simulink model "OilWellDrillingTesting"  (R2021a)
settings: Solver=ode4  StartTime=0.0  StopTime=4800  FixedStep=0.1  RelTol=1e-3
libraries: simulink x1
settings Model: Creator=isak.skeie  LastModifiedBy=isak.skeie

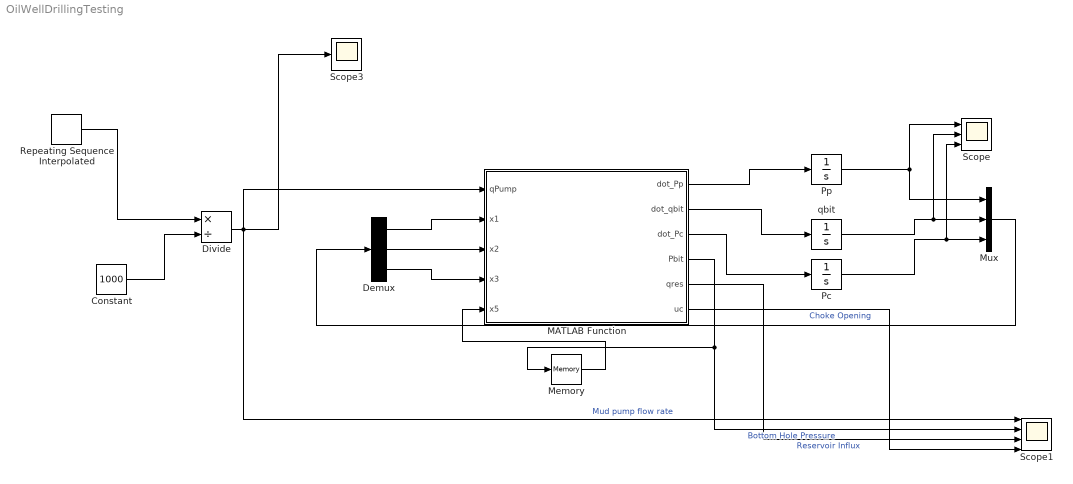
== system OilWellDrillingTesting ==
  Constant : Constant  Value=1000
  Demux : Demux  Outputs=3
  Divide : Product  Inputs=*/
  MATLAB Function : MATLAB Function  TreatAsAtomicUnit=on
  Memory : Memory
  Mux : Mux  Inputs=3
  Pc : Integrator  InitialCondition=5*10^5
  Pp : Integrator  InitialCondition=8*10^5
  Repeating Sequence Interpolated : simulink/Sources/Repeating Sequence Interpolated  OutValues="[25 25  0 0  25 25 0 0 25 25].'"  TimeValues=[0 600 900 1500 1800 2700 3000 3600 3900 4800].'  LookUpMeth=Interpolation-Use End Values  tsamp=0.1  OutMin=[0]  OutMax=[0.025]  OutDataTypeStr=double  OutputDataTypeScalingMode=double  OutDataType=fixdt(0,8)  OutScaling=2^-10
  Scope : Scope  NumInputPorts=3
  Scope1 : Scope  NumInputPorts=4
  Scope3 : Scope
  qbit : Integrator  InitialCondition=0.025
  wires:
  MATLAB Function/1(dot_Pp) -> Pp/1
  MATLAB Function/2(dot_qbit) -> qbit/1
  MATLAB Function/3(dot_Pc) -> Pc/1
  Pp/1 -> Mux/1, Scope/1
  qbit/1 -> Scope/2, Mux/2
  Pc/1 -> Scope/3, Mux/3
  Demux/1 -> MATLAB Function/2(x1)
  Demux/2 -> MATLAB Function/3(x2)
  Demux/3 -> MATLAB Function/4(x3)
  Mux/1 -> Demux/1
  MATLAB Function/4(Pbit) -> Scope1/2, Memory/1  "Bottom Hole Pressure"
  Memory/1 -> MATLAB Function/5(x5)
  Repeating Sequence Interpolated/1 -> Divide/1
  Constant/1 -> Divide/2
  Divide/1 -> Scope1/1, MATLAB Function/1(qPump), Scope3/1  "Mud pump flow rate"
  MATLAB Function/5(qres) -> Scope1/3  "Reservoir Influx"
  MATLAB Function/6(uc) -> Scope1/4  "Choke Opening"

== matlab function OilWellDrillingTesting/MATLAB Function ==
  data: qPump input; x1 input; dot_Pp output; x2 input; x3 input; dot_qbit output; dot_Pc output; Pbit output; qres output; x5 input; uc output
function [dot_Pp, dot_qbit, dot_Pc,Pbit, qres, uc] = OilWell(qPump, x1, x2, x3, x5)

%States
Pp = x1;
qbit = x2;
Pc = x3;
Pbit = x5
%input
qpump = qPump;


%Parameters

pl  = 1150;              %kg/m^3    Drill mud density
pw  = 1000;              %kg/m^3    Water Density
WC  = 0.1;               %          Water cut of the reservoir fluid
Ad  = 0.0067;            %m^2       Cross sectional area of drilling string
Aa  = 0.278;             %m^2       Cross sectional area of annulus
Dd  = 0.0925;            %m         Hydraulic diameter of drill string
Da  = 0.211;             %m         Hydraulic diameter of annulus
L   = 1600.0;            %m         Vertical depth of the well
PI  = 1.6667*10^(-9);    %m^5/Ns    Productivity Index Value          
Pres = 250*10^5;         %N/m^2     Reservoir pressure
Pfrac = 270*10^5;        %N/m^2     Fracture pressure
Pcoll = 220*10^5;        %N/m^2     Collapse pressure
Prefbit = 0;             %N/m^2     Reference pressure 
P0  =  4*10^5;           %N/m^2     Pressure downstream the choke valve
eDd = 10^(-5);           %Relative roughness of pipe in drill string
eDa = 10^(-4);           %Relative roughness of pipe in the annulus
ud = 0.015;              %kg/ms     Dynamic viscosity of the drill fluid
bd = 3*10^8;             %N/m^2     Bulk modulus in the drill string
ba = 2.4*10^8;           %N/m^2     Bulk modulus in the annulus
qnom = 1500;             %l/min     Nominal flow rate of the drill fluid
uc = 70;                 %%         Nominal choke valve opening
g = 9.81;                %m/s^2     Acceleration due to gravity
fd = 0.02;               %          Friction factor




%Declare Process Variables
%deltaP_df = 0;           %N/m^2      Pressure difference due to friction drill string   
%deltaP_af = 0;           %N/m^2      Pressure difference due to friction in annulus
%Pbit = 0;                %N/m^2      Bottom hole pressure 
%qres = 0;                %m^3/s      Flow rate of reservoir fluid
qback = 0;               %m^3/s      Flow rate of Back pressure pump
%qchoke = 0;              %m^3/s      Flow rate through choke valve
 
              
pmix     = pw*WC + (1 - WC)*pl;                          %Density of fluid in annulus     !! qres = 0 then WX = 0
  
N6 = 27.3 / (3600*sqrt(10^5));
Zc = 0;                 %Valve characteristics as function of opening

if uc < 5              
    Zc = 0;
elseif (5 <= uc) && uc < 50
    Zc = 0.111*uc - 0.556;
elseif uc >= 50
     Zc = 0.5*uc - 20;
end




%Functions
 qres     = max(PI*(Pres - Pbit),0); 
 va = (qbit+qres)/( Aa); 
 deltaP_af = (fd*L*pmix*va^2)/(2*Da);
 Pbit     = Pc + pmix*g*L + deltaP_af;                    %Bottom hole pressure   
                              %Flow rate into Annulus
 vd = qpump/(Ad);                                        %Drill string velocity
                                 %Annulus velocity
 deltaP_df = (fd*L*pl*vd^2)/(2*Dd);                      %Pressure difference due to friction drill string 
  
 
 %Conditions
     
if qres == 0
     WX = 0;
end


if Pc < P0
     qchoke = 0;
else 
     qchoke   = N6*Zc*sqrt((Pc-P0)/pmix);                     %Flow rate through choke valve, Do MAX??
end



dot_L    = 0;  



%Differential equations
  
  dot_Pp   = (bd/(Ad*L))*(qpump - qbit);                   %N/m^2/s    Well head pressure change
  dot_qbit = (Ad/(pl*L))*(Pp + pl*g*L - deltaP_df - Pbit); %m^3/s      Flow rate through drill bit
  dot_Pc   = (ba/(Aa*L))*(qbit + qres + qback - qchoke);   %N/m^2/s    Change in pressure at annulus head

  

 %Conditions
if qbit <= 0 & dot_qbit < 0
    dot_qbit = 0;
    qbit = 0
end
